simulink model "espectro"  (R2012b)
settings: Solver=ode45  StartTime=0.0  StopTime=10.0  RelTol=1e-3
libraries: xbsIndex_r4 x39, xps_library x25, dspsigops x16, monroe_library x2
settings Model: Creator=root  LastModifiedBy=root

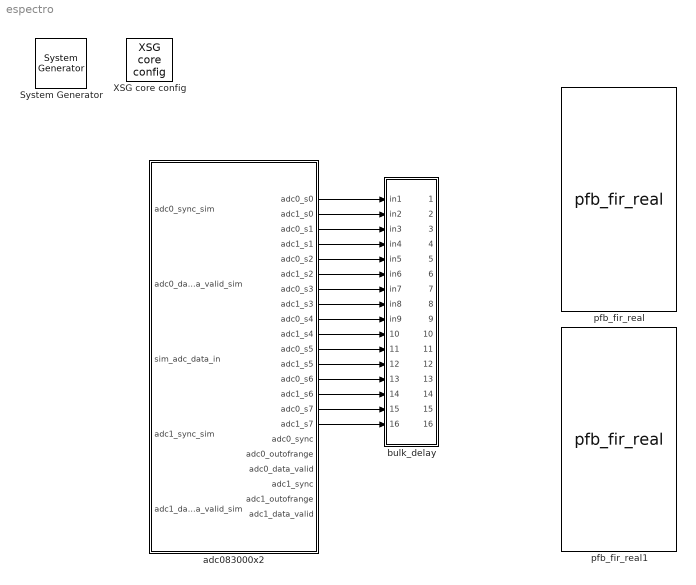
== system espectro ==
  " System Generator" : xbsIndex_r4/ System Generator  Tag=genX  xilinxfamily=virtex5  part=xc5vsx95t  speed=-1  package=ff1136  synthesis_tool=XST  clock_wrapper=Clock Enables  directory=./spec_2pol_4kw_6tap_pfb/sysgen  proj_type=Project Navigator  Synth_file=XST Defaults  Impl_file=ISE Defaults  testbench=off  simulink_period=1  sysclk_period=2.6667  dcm_input_clock_period=100  incr_netlist=off  trim_vbits=Everywhere in SubSystem  dbl_ovrd=According to Block Masks  core_generation=According to Block Masks  run_coregen=off  deprecated_control=off  eval_field=0  block_type=sysgen
      settings: block_version=11.4
  XSG core config : xps_library/XSG core config  Tag=xps:xsg  hw_sys=ROACH:sx95t  clk_src=adc0_clk  ROACH_clk_src=adc0_clk  ROACH2_clk_src=adc0_clk  clk_rate=375  sample_period=1  synthesis_tool=XST
  adc083000x2 : Subsystem  Tag=xps:adc083000x2  AncestorBlock=xps_library/adc083000x2  mask(adc_083000x2){use_adc0=on, use_adc1=on, demux_adc=off, clock_sync=on, verbose=off, using_ctrl=on, adc_clk_rate=1000, sample_period=1, bit_width=8}
      mask prompts: use_adc0 "Use ZD0K0?"; use_adc1 "Use ZDOK1?"; demux_adc "Demux ADCs by 2?"; clock_sync "Interleave 2 ADC boards?"; verbose "Verbose Block Creation?"; using_ctrl "Add ports for control registers?"; adc_clk_rate "ADC clock rate (MHz)"; sample_period "Sample Period"; bit_width "Output Bit Width"
      mask help:
      | The ADC block converts analog inputs to digital outputs.
      | Every clock cycle, the inputs are sampled and digitized to
      | 8 bit binary point numbers in the range of [-1, 1).
      |
      | Online block-specific documentation: http://casper.berkeley.edu/wiki/Adc083000
      mask init:
      | adc083000_mask;
      mask Help: eval('xlWeb([getenv(''MLIB_ROOT''), ''\doc\html\sys_adc\sys_adc.html''])')
  bulk_delay : Subsystem  AncestorBlock=monroe_library/bulk_delay  mask{numInputs=9, delay_arr=5}
      mask prompts: numInputs "# Inputs?"; delay_arr "Delays (integer or array of #inputs elements)"
      mask init:
      | config.source=str2func('bulk_delay_draw');
      | config.toplevel=gcb;
      | config.debug=0;
      | config.depend={'bulk_delay_draw.m'};
      | xBlock(config,{numInputs,delay_arr});
  pfb_fir_real : monroe_library/pfb_fir_real  pfb_size=14  n_sim_inputs=4  n_taps=4  data_n_bits=18  coeff_n_bits=18  output_bit_width=18  window_fn=hamming  bin_width=1  end_scale_val=1  endDelay=off  cheap_sync=off  autoplace_mode='Attached to both ADC0 and ADC1 (interleaved)'  autoplace_optimize=off  bram_latency_coeff=off  bram_latency_delay=off  register_counter=off  pack_delays=on
  pfb_fir_real1 : monroe_library/pfb_fir_real  pfb_size=14  n_sim_inputs=4  n_taps=4  data_n_bits=18  coeff_n_bits=18  output_bit_width=18  window_fn=hamming  bin_width=1  end_scale_val=1  endDelay=off  cheap_sync=off  autoplace_mode='Attached to both ADC0 and ADC1 (interleaved)'  autoplace_optimize=off  bram_latency_coeff=off  bram_latency_delay=off  register_counter=off  pack_delays=on
  wires:
  adc083000x2/1(adc0_s0) -> bulk_delay/1(in1)
  adc083000x2/2(adc1_s0) -> bulk_delay/2(in2)
  adc083000x2/3(adc0_s1) -> bulk_delay/3(in3)
  adc083000x2/4(adc1_s1) -> bulk_delay/4(in4)
  adc083000x2/5(adc0_s2) -> bulk_delay/5(in5)
  adc083000x2/6(adc1_s2) -> bulk_delay/6(in6)
  adc083000x2/7(adc0_s3) -> bulk_delay/7(in7)
  adc083000x2/8(adc1_s3) -> bulk_delay/8(in8)
  adc083000x2/9(adc0_s4) -> bulk_delay/9(in9)
  adc083000x2/10(adc1_s4) -> bulk_delay/10(in10)
  adc083000x2/11(adc0_s5) -> bulk_delay/11(in11)
  adc083000x2/12(adc1_s5) -> bulk_delay/12(in12)
  adc083000x2/13(adc0_s6) -> bulk_delay/13(in13)
  adc083000x2/14(adc1_s6) -> bulk_delay/14(in14)
  adc083000x2/15(adc0_s7) -> bulk_delay/15(in15)
  adc083000x2/16(adc1_s7) -> bulk_delay/16(in16)

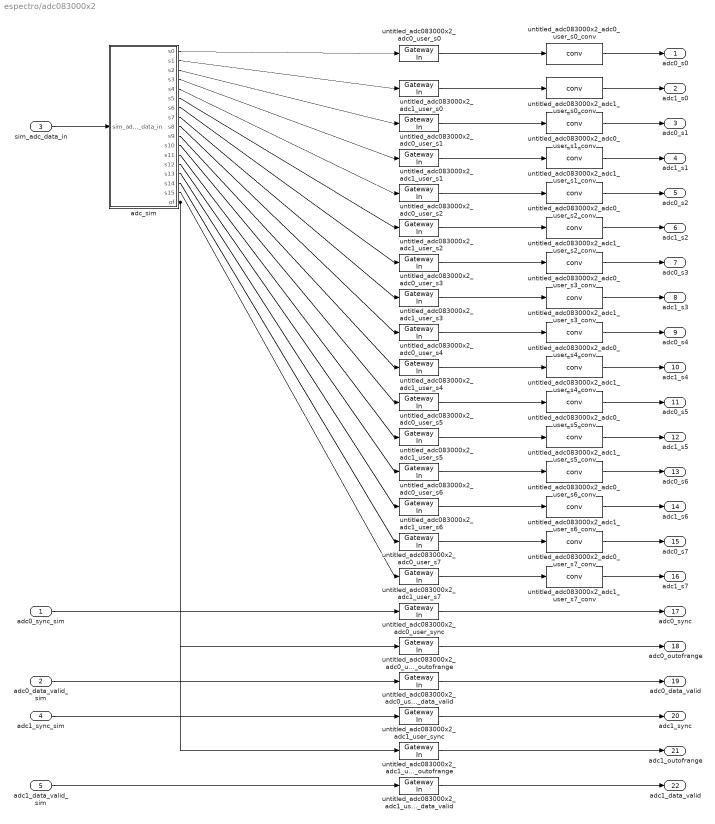
== system espectro/adc083000x2 ==
  adc0_sync_sim : Inport
  adc0_data_valid_sim : Inport  Port=2
  sim_adc_data_in : Inport  Port=3
  adc1_sync_sim : Inport  Port=4
  adc1_data_valid_sim : Inport  Port=5
  adc_sim : Subsystem  AncestorBlock=xps_library/ADCs/adc_sim  mask(adc_sim){nStreams=16, bit_width=8}
      mask prompts: nStreams "Number of Output Streams"; bit_width "Sample Bit Width"
      mask help:
      | This block simulates the behavior of a demuxed ADC, which takes
      | as input a waveform and returns digital samples in parallel at
      | a slower rate.
      |
      | This block is used to simulate the behavior
      mask init:
      | adc_sim_init(gcb, ...
      |     'nStreams', nStreams, ...
      |     'bit_width', bit_width);
  untitled_adc083000x2_adc0_user_data_valid : xbsIndex_r4/Gateway In  gui_display_data_type=Fixed-point  arith_type=Unsigned  n_bits=1  bin_pt=0  preci_type=Single  exp_width=8  frac_width=24  quantization="Round  (unbiased: +/- Inf)"  overflow=Saturate  period=1  dbl_ovrd=off  timing_constraint=None  locs_specified=off  LOCs={}  UseAsADC=off  ADCChannel='1'  inherit_from_input=off  hdl_port=on  block_type=gatewayin
  untitled_adc083000x2_adc0_user_outofrange : xbsIndex_r4/Gateway In  gui_display_data_type=Fixed-point  arith_type=Unsigned  n_bits=4  bin_pt=0  preci_type=Single  exp_width=8  frac_width=24  quantization="Round  (unbiased: +/- Inf)"  overflow=Saturate  period=1  dbl_ovrd=off  timing_constraint=None  locs_specified=off  LOCs={}  UseAsADC=off  ADCChannel='1'  inherit_from_input=off  hdl_port=on  block_type=gatewayin
  untitled_adc083000x2_adc0_user_s{0..7} (8 alike) : xbsIndex_r4/Gateway In  gui_display_data_type=Fixed-point  arith_type=Unsigned  n_bits=8  bin_pt=0  preci_type=Single  exp_width=8  frac_width=24  quantization="Round  (unbiased: +/- Inf)"  overflow=Saturate  period=1  dbl_ovrd=off  timing_constraint=None  locs_specified=off  LOCs={}  UseAsADC=off  ADCChannel='1'  inherit_from_input=off  hdl_port=on  block_type=gatewayin
  untitled_adc083000x2_adc0_user_s0_conv : xps_library/ADCs/conv  bit_width=8
  untitled_adc083000x2_adc0_user_s1_conv : xps_library/ADCs/conv  bit_width=8
  untitled_adc083000x2_adc0_user_s2_conv : xps_library/ADCs/conv  bit_width=8
  untitled_adc083000x2_adc0_user_s3_conv : xps_library/ADCs/conv  bit_width=8
  untitled_adc083000x2_adc0_user_s4_conv : xps_library/ADCs/conv  bit_width=8
  untitled_adc083000x2_adc0_user_s5_conv : xps_library/ADCs/conv  bit_width=8
  untitled_adc083000x2_adc0_user_s6_conv : xps_library/ADCs/conv  bit_width=8
  untitled_adc083000x2_adc0_user_s7_conv : xps_library/ADCs/conv  bit_width=8
  untitled_adc083000x2_adc0_user_sync : xbsIndex_r4/Gateway In  gui_display_data_type=Fixed-point  arith_type=Unsigned  n_bits=4  bin_pt=0  preci_type=Single  exp_width=8  frac_width=24  quantization="Round  (unbiased: +/- Inf)"  overflow=Saturate  period=1  dbl_ovrd=off  timing_constraint=None  locs_specified=off  LOCs={}  UseAsADC=off  ADCChannel='1'  inherit_from_input=off  hdl_port=on  block_type=gatewayin
  untitled_adc083000x2_adc1_user_data_valid : xbsIndex_r4/Gateway In  gui_display_data_type=Fixed-point  arith_type=Unsigned  n_bits=1  bin_pt=0  preci_type=Single  exp_width=8  frac_width=24  quantization="Round  (unbiased: +/- Inf)"  overflow=Saturate  period=1  dbl_ovrd=off  timing_constraint=None  locs_specified=off  LOCs={}  UseAsADC=off  ADCChannel='1'  inherit_from_input=off  hdl_port=on  block_type=gatewayin
  untitled_adc083000x2_adc1_user_outofrange : xbsIndex_r4/Gateway In  gui_display_data_type=Fixed-point  arith_type=Unsigned  n_bits=4  bin_pt=0  preci_type=Single  exp_width=8  frac_width=24  quantization="Round  (unbiased: +/- Inf)"  overflow=Saturate  period=1  dbl_ovrd=off  timing_constraint=None  locs_specified=off  LOCs={}  UseAsADC=off  ADCChannel='1'  inherit_from_input=off  hdl_port=on  block_type=gatewayin
  untitled_adc083000x2_adc1_user_s{0..7} (8 alike) : xbsIndex_r4/Gateway In  gui_display_data_type=Fixed-point  arith_type=Unsigned  n_bits=8  bin_pt=0  preci_type=Single  exp_width=8  frac_width=24  quantization="Round  (unbiased: +/- Inf)"  overflow=Saturate  period=1  dbl_ovrd=off  timing_constraint=None  locs_specified=off  LOCs={}  UseAsADC=off  ADCChannel='1'  inherit_from_input=off  hdl_port=on  block_type=gatewayin
  untitled_adc083000x2_adc1_user_s0_conv : xps_library/ADCs/conv  bit_width=8
  untitled_adc083000x2_adc1_user_s1_conv : xps_library/ADCs/conv  bit_width=8
  untitled_adc083000x2_adc1_user_s2_conv : xps_library/ADCs/conv  bit_width=8
  untitled_adc083000x2_adc1_user_s3_conv : xps_library/ADCs/conv  bit_width=8
  untitled_adc083000x2_adc1_user_s4_conv : xps_library/ADCs/conv  bit_width=8
  untitled_adc083000x2_adc1_user_s5_conv : xps_library/ADCs/conv  bit_width=8
  untitled_adc083000x2_adc1_user_s6_conv : xps_library/ADCs/conv  bit_width=8
  untitled_adc083000x2_adc1_user_s7_conv : xps_library/ADCs/conv  bit_width=8
  untitled_adc083000x2_adc1_user_sync : xbsIndex_r4/Gateway In  gui_display_data_type=Fixed-point  arith_type=Unsigned  n_bits=4  bin_pt=0  preci_type=Single  exp_width=8  frac_width=24  quantization="Round  (unbiased: +/- Inf)"  overflow=Saturate  period=1  dbl_ovrd=off  timing_constraint=None  locs_specified=off  LOCs={}  UseAsADC=off  ADCChannel='1'  inherit_from_input=off  hdl_port=on  block_type=gatewayin
  adc0_s0 : Outport
  adc1_s0 : Outport  Port=2
  adc0_s1 : Outport  Port=3
  adc1_s1 : Outport  Port=4
  adc0_s2 : Outport  Port=5
  adc1_s2 : Outport  Port=6
  adc0_s3 : Outport  Port=7
  adc1_s3 : Outport  Port=8
  adc0_s4 : Outport  Port=9
  adc1_s4 : Outport  Port=10
  adc0_s5 : Outport  Port=11
  adc1_s5 : Outport  Port=12
  adc0_s6 : Outport  Port=13
  adc1_s6 : Outport  Port=14
  adc0_s7 : Outport  Port=15
  adc1_s7 : Outport  Port=16
  adc0_sync : Outport  Port=17
  adc0_outofrange : Outport  Port=18
  adc0_data_valid : Outport  Port=19
  adc1_sync : Outport  Port=20
  adc1_outofrange : Outport  Port=21
  adc1_data_valid : Outport  Port=22
  wires:
  sim_adc_data_in/1 -> adc_sim/1(sim_adc_data_in)
  adc_sim/1(s0) -> untitled_adc083000x2_adc0_user_s0/1
  untitled_adc083000x2_adc0_user_s0/1 -> untitled_adc083000x2_adc0_user_s0_conv/1
  untitled_adc083000x2_adc0_user_s0_conv/1 -> adc0_s0/1
  adc_sim/2(s1) -> untitled_adc083000x2_adc1_user_s0/1
  untitled_adc083000x2_adc1_user_s0/1 -> untitled_adc083000x2_adc1_user_s0_conv/1
  untitled_adc083000x2_adc1_user_s0_conv/1 -> adc1_s0/1
  adc_sim/3(s2) -> untitled_adc083000x2_adc0_user_s1/1
  untitled_adc083000x2_adc0_user_s1/1 -> untitled_adc083000x2_adc0_user_s1_conv/1
  untitled_adc083000x2_adc0_user_s1_conv/1 -> adc0_s1/1
  adc_sim/4(s3) -> untitled_adc083000x2_adc1_user_s1/1
  untitled_adc083000x2_adc1_user_s1/1 -> untitled_adc083000x2_adc1_user_s1_conv/1
  untitled_adc083000x2_adc1_user_s1_conv/1 -> adc1_s1/1
  adc_sim/5(s4) -> untitled_adc083000x2_adc0_user_s2/1
  untitled_adc083000x2_adc0_user_s2/1 -> untitled_adc083000x2_adc0_user_s2_conv/1
  untitled_adc083000x2_adc0_user_s2_conv/1 -> adc0_s2/1
  adc_sim/6(s5) -> untitled_adc083000x2_adc1_user_s2/1
  untitled_adc083000x2_adc1_user_s2/1 -> untitled_adc083000x2_adc1_user_s2_conv/1
  untitled_adc083000x2_adc1_user_s2_conv/1 -> adc1_s2/1
  adc_sim/7(s6) -> untitled_adc083000x2_adc0_user_s3/1
  untitled_adc083000x2_adc0_user_s3/1 -> untitled_adc083000x2_adc0_user_s3_conv/1
  untitled_adc083000x2_adc0_user_s3_conv/1 -> adc0_s3/1
  adc_sim/8(s7) -> untitled_adc083000x2_adc1_user_s3/1
  untitled_adc083000x2_adc1_user_s3/1 -> untitled_adc083000x2_adc1_user_s3_conv/1
  untitled_adc083000x2_adc1_user_s3_conv/1 -> adc1_s3/1
  adc_sim/9(s8) -> untitled_adc083000x2_adc0_user_s4/1
  untitled_adc083000x2_adc0_user_s4/1 -> untitled_adc083000x2_adc0_user_s4_conv/1
  untitled_adc083000x2_adc0_user_s4_conv/1 -> adc0_s4/1
  adc_sim/10(s9) -> untitled_adc083000x2_adc1_user_s4/1
  untitled_adc083000x2_adc1_user_s4/1 -> untitled_adc083000x2_adc1_user_s4_conv/1
  untitled_adc083000x2_adc1_user_s4_conv/1 -> adc1_s4/1
  adc_sim/11(s10) -> untitled_adc083000x2_adc0_user_s5/1
  untitled_adc083000x2_adc0_user_s5/1 -> untitled_adc083000x2_adc0_user_s5_conv/1
  untitled_adc083000x2_adc0_user_s5_conv/1 -> adc0_s5/1
  adc_sim/12(s11) -> untitled_adc083000x2_adc1_user_s5/1
  untitled_adc083000x2_adc1_user_s5/1 -> untitled_adc083000x2_adc1_user_s5_conv/1
  untitled_adc083000x2_adc1_user_s5_conv/1 -> adc1_s5/1
  adc_sim/13(s12) -> untitled_adc083000x2_adc0_user_s6/1
  untitled_adc083000x2_adc0_user_s6/1 -> untitled_adc083000x2_adc0_user_s6_conv/1
  untitled_adc083000x2_adc0_user_s6_conv/1 -> adc0_s6/1
  adc_sim/14(s13) -> untitled_adc083000x2_adc1_user_s6/1
  untitled_adc083000x2_adc1_user_s6/1 -> untitled_adc083000x2_adc1_user_s6_conv/1
  untitled_adc083000x2_adc1_user_s6_conv/1 -> adc1_s6/1
  adc_sim/15(s14) -> untitled_adc083000x2_adc0_user_s7/1
  untitled_adc083000x2_adc0_user_s7/1 -> untitled_adc083000x2_adc0_user_s7_conv/1
  untitled_adc083000x2_adc0_user_s7_conv/1 -> adc0_s7/1
  adc_sim/16(s15) -> untitled_adc083000x2_adc1_user_s7/1
  untitled_adc083000x2_adc1_user_s7/1 -> untitled_adc083000x2_adc1_user_s7_conv/1
  untitled_adc083000x2_adc1_user_s7_conv/1 -> adc1_s7/1
  adc0_sync_sim/1 -> untitled_adc083000x2_adc0_user_sync/1
  untitled_adc083000x2_adc0_user_sync/1 -> adc0_sync/1
  adc_sim/17(of) -> untitled_adc083000x2_adc0_user_outofrange/1, untitled_adc083000x2_adc1_user_outofrange/1
  untitled_adc083000x2_adc0_user_outofrange/1 -> adc0_outofrange/1
  adc0_data_valid_sim/1 -> untitled_adc083000x2_adc0_user_data_valid/1
  untitled_adc083000x2_adc0_user_data_valid/1 -> adc0_data_valid/1
  adc1_sync_sim/1 -> untitled_adc083000x2_adc1_user_sync/1
  untitled_adc083000x2_adc1_user_sync/1 -> adc1_sync/1
  untitled_adc083000x2_adc1_user_outofrange/1 -> adc1_outofrange/1
  adc1_data_valid_sim/1 -> untitled_adc083000x2_adc1_user_data_valid/1
  untitled_adc083000x2_adc1_user_data_valid/1 -> adc1_data_valid/1

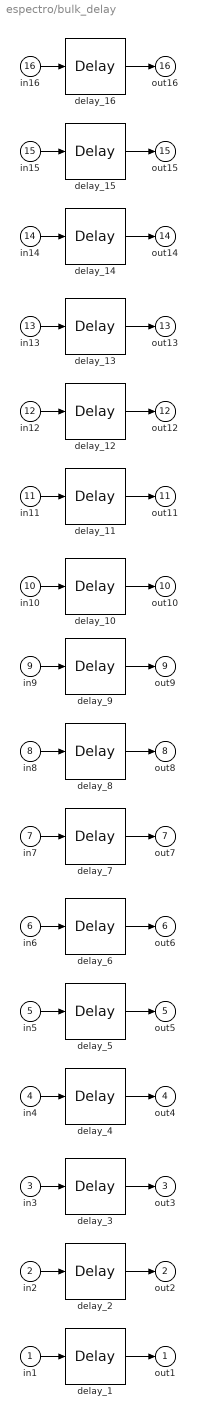
== system espectro/bulk_delay ==
  in1 : Inport
  in2 : Inport  Port=2
  in3 : Inport  Port=3
  in4 : Inport  Port=4
  in5 : Inport  Port=5
  in6 : Inport  Port=6
  in7 : Inport  Port=7
  in8 : Inport  Port=8
  in9 : Inport  Port=9
  in10 : Inport  Port=10
  in11 : Inport  Port=11
  in12 : Inport  Port=12
  in13 : Inport  Port=13
  in14 : Inport  Port=14
  in15 : Inport  Port=15
  in16 : Inport  Port=16
  delay_{1..16} (16 alike) : xbsIndex_r4/Delay  rst=off  infoeditControl=Selection of Reset will increase slice count due to use of real FFs and instead of SRLs  en=off  latency=5  dbl_ovrd=off  reg_retiming=off  block_type=delay
  out1 : Outport
  out2 : Outport  Port=2
  out3 : Outport  Port=3
  out4 : Outport  Port=4
  out5 : Outport  Port=5
  out6 : Outport  Port=6
  out7 : Outport  Port=7
  out8 : Outport  Port=8
  out9 : Outport  Port=9
  out10 : Outport  Port=10
  out11 : Outport  Port=11
  out12 : Outport  Port=12
  out13 : Outport  Port=13
  out14 : Outport  Port=14
  out15 : Outport  Port=15
  out16 : Outport  Port=16
  wires:
  in1/1 -> delay_1/1
  delay_1/1 -> out1/1
  in2/1 -> delay_2/1
  delay_2/1 -> out2/1
  in3/1 -> delay_3/1
  delay_3/1 -> out3/1
  in4/1 -> delay_4/1
  delay_4/1 -> out4/1
  in5/1 -> delay_5/1
  delay_5/1 -> out5/1
  in6/1 -> delay_6/1
  delay_6/1 -> out6/1
  in7/1 -> delay_7/1
  delay_7/1 -> out7/1
  in8/1 -> delay_8/1
  delay_8/1 -> out8/1
  in9/1 -> delay_9/1
  delay_9/1 -> out9/1
  in10/1 -> delay_10/1
  delay_10/1 -> out10/1
  in11/1 -> delay_11/1
  delay_11/1 -> out11/1
  in12/1 -> delay_12/1
  delay_12/1 -> out12/1
  in13/1 -> delay_13/1
  delay_13/1 -> out13/1
  in14/1 -> delay_14/1
  delay_14/1 -> out14/1
  in15/1 -> delay_15/1
  delay_15/1 -> out15/1
  in16/1 -> delay_16/1
  delay_16/1 -> out16/1

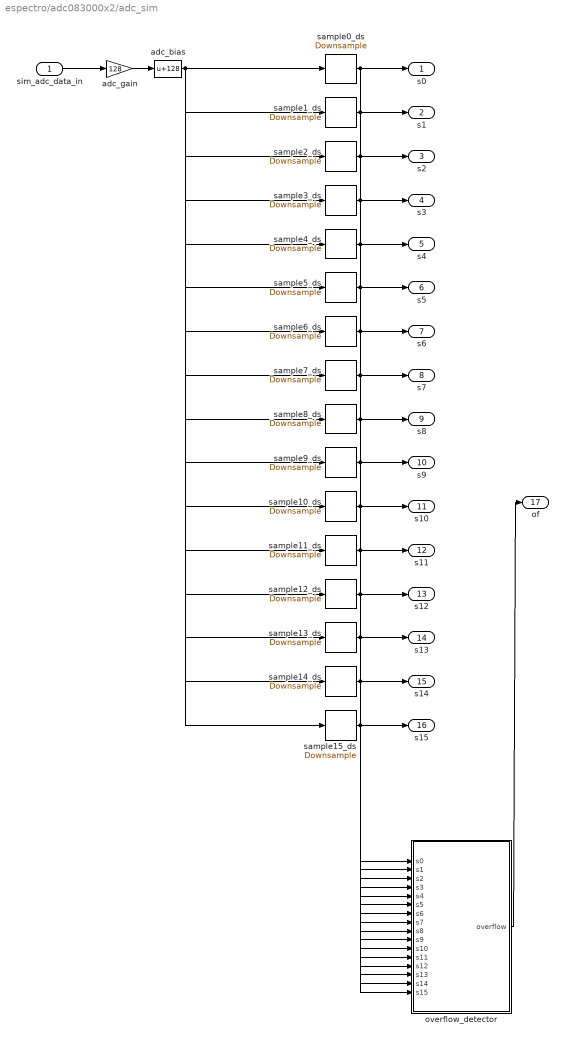
== system espectro/adc083000x2/adc_sim ==
  sim_adc_data_in : Inport
  adc_bias : Bias  Bias=128  SaturateOnIntegerOverflow=on
  adc_gain : Gain  Gain=128
  overflow_detector : Subsystem  AncestorBlock=xps_library/ADCs/of_detect_bus  mask(of_detect_bus){nStreams=16, bit_width=8}
      mask prompts: nStreams "Number of Streams"; bit_width "Bit Width"
      mask init:
      | of_detect_bus_init(gcb, ...
      |     'nStreams', nStreams, ...
      |     'bit_width', bit_width);
  sample0_ds : dspsigops/Downsample  N=16  phase=1  InputProcessing=Inherited (this choice will be removed - see release notes)  RateOptions=Enforce single-rate processing  smode=Force single rate  fmode=Maintain input frame rate  ic=0
  sample10_ds : dspsigops/Downsample  N=16  phase=11  InputProcessing=Inherited (this choice will be removed - see release notes)  RateOptions=Enforce single-rate processing  smode=Force single rate  fmode=Maintain input frame rate  ic=0
  sample11_ds : dspsigops/Downsample  N=16  phase=12  InputProcessing=Inherited (this choice will be removed - see release notes)  RateOptions=Enforce single-rate processing  smode=Force single rate  fmode=Maintain input frame rate  ic=0
  sample12_ds : dspsigops/Downsample  N=16  phase=13  InputProcessing=Inherited (this choice will be removed - see release notes)  RateOptions=Enforce single-rate processing  smode=Force single rate  fmode=Maintain input frame rate  ic=0
  sample13_ds : dspsigops/Downsample  N=16  phase=14  InputProcessing=Inherited (this choice will be removed - see release notes)  RateOptions=Enforce single-rate processing  smode=Force single rate  fmode=Maintain input frame rate  ic=0
  sample14_ds : dspsigops/Downsample  N=16  phase=15  InputProcessing=Inherited (this choice will be removed - see release notes)  RateOptions=Enforce single-rate processing  smode=Force single rate  fmode=Maintain input frame rate  ic=0
  sample15_ds : dspsigops/Downsample  N=16  phase=0  InputProcessing=Inherited (this choice will be removed - see release notes)  RateOptions=Enforce single-rate processing  smode=Force single rate  fmode=Maintain input frame rate  ic=0
  sample1_ds : dspsigops/Downsample  N=16  phase=2  InputProcessing=Inherited (this choice will be removed - see release notes)  RateOptions=Enforce single-rate processing  smode=Force single rate  fmode=Maintain input frame rate  ic=0
  sample2_ds : dspsigops/Downsample  N=16  phase=3  InputProcessing=Inherited (this choice will be removed - see release notes)  RateOptions=Enforce single-rate processing  smode=Force single rate  fmode=Maintain input frame rate  ic=0
  sample3_ds : dspsigops/Downsample  N=16  phase=4  InputProcessing=Inherited (this choice will be removed - see release notes)  RateOptions=Enforce single-rate processing  smode=Force single rate  fmode=Maintain input frame rate  ic=0
  sample4_ds : dspsigops/Downsample  N=16  phase=5  InputProcessing=Inherited (this choice will be removed - see release notes)  RateOptions=Enforce single-rate processing  smode=Force single rate  fmode=Maintain input frame rate  ic=0
  sample5_ds : dspsigops/Downsample  N=16  phase=6  InputProcessing=Inherited (this choice will be removed - see release notes)  RateOptions=Enforce single-rate processing  smode=Force single rate  fmode=Maintain input frame rate  ic=0
  sample6_ds : dspsigops/Downsample  N=16  phase=7  InputProcessing=Inherited (this choice will be removed - see release notes)  RateOptions=Enforce single-rate processing  smode=Force single rate  fmode=Maintain input frame rate  ic=0
  sample7_ds : dspsigops/Downsample  N=16  phase=8  InputProcessing=Inherited (this choice will be removed - see release notes)  RateOptions=Enforce single-rate processing  smode=Force single rate  fmode=Maintain input frame rate  ic=0
  sample8_ds : dspsigops/Downsample  N=16  phase=9  InputProcessing=Inherited (this choice will be removed - see release notes)  RateOptions=Enforce single-rate processing  smode=Force single rate  fmode=Maintain input frame rate  ic=0
  sample9_ds : dspsigops/Downsample  N=16  phase=10  InputProcessing=Inherited (this choice will be removed - see release notes)  RateOptions=Enforce single-rate processing  smode=Force single rate  fmode=Maintain input frame rate  ic=0
  s0 : Outport
  s1 : Outport  Port=2
  s2 : Outport  Port=3
  s3 : Outport  Port=4
  s4 : Outport  Port=5
  s5 : Outport  Port=6
  s6 : Outport  Port=7
  s7 : Outport  Port=8
  s8 : Outport  Port=9
  s9 : Outport  Port=10
  s10 : Outport  Port=11
  s11 : Outport  Port=12
  s12 : Outport  Port=13
  s13 : Outport  Port=14
  s14 : Outport  Port=15
  s15 : Outport  Port=16
  of : Outport  Port=17
  wires:
  sim_adc_data_in/1 -> adc_gain/1
  adc_gain/1 -> adc_bias/1
  overflow_detector/1(overflow) -> of/1
  adc_bias/1 -> sample0_ds/1, sample1_ds/1, sample2_ds/1, sample3_ds/1, sample4_ds/1, sample5_ds/1, sample6_ds/1, sample7_ds/1, sample8_ds/1, sample9_ds/1, sample10_ds/1, sample11_ds/1, sample12_ds/1, sample13_ds/1, sample14_ds/1, sample15_ds/1
  sample0_ds/1 -> overflow_detector/1(s0), s0/1
  sample1_ds/1 -> overflow_detector/2(s1), s1/1
  sample2_ds/1 -> overflow_detector/3(s2), s2/1
  sample3_ds/1 -> overflow_detector/4(s3), s3/1
  sample4_ds/1 -> overflow_detector/5(s4), s4/1
  sample5_ds/1 -> overflow_detector/6(s5), s5/1
  sample6_ds/1 -> overflow_detector/7(s6), s6/1
  sample7_ds/1 -> overflow_detector/8(s7), s7/1
  sample8_ds/1 -> overflow_detector/9(s8), s8/1
  sample9_ds/1 -> overflow_detector/10(s9), s9/1
  sample10_ds/1 -> overflow_detector/11(s10), s10/1
  sample11_ds/1 -> overflow_detector/12(s11), s11/1
  sample12_ds/1 -> overflow_detector/13(s12), s12/1
  sample13_ds/1 -> overflow_detector/14(s13), s13/1
  sample14_ds/1 -> overflow_detector/15(s14), s14/1
  sample15_ds/1 -> overflow_detector/16(s15), s15/1

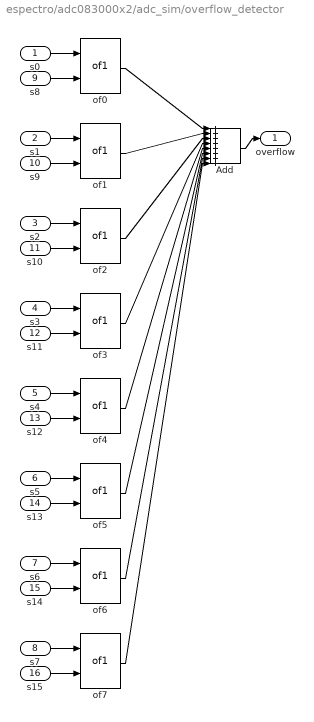
== system espectro/adc083000x2/adc_sim/overflow_detector ==
  s0 : Inport
  s1 : Inport  Port=2
  s2 : Inport  Port=3
  s3 : Inport  Port=4
  s4 : Inport  Port=5
  s5 : Inport  Port=6
  s6 : Inport  Port=7
  s7 : Inport  Port=8
  s8 : Inport  Port=9
  s9 : Inport  Port=10
  s10 : Inport  Port=11
  s11 : Inport  Port=12
  s12 : Inport  Port=13
  s13 : Inport  Port=14
  s14 : Inport  Port=15
  s15 : Inport  Port=16
  Add : Sum  Inputs=++++++++
  of{0..7} (8 alike) : xps_library/ADCs/of1  bit_num=0  n_adc_bits=8
  overflow : Outport
  wires:
  s0/1 -> of0/1
  s8/1 -> of0/2
  of0/1 -> Add/1
  s1/1 -> of1/1
  s9/1 -> of1/2
  of1/1 -> Add/2
  s2/1 -> of2/1
  s10/1 -> of2/2
  of2/1 -> Add/3
  s3/1 -> of3/1
  s11/1 -> of3/2
  of3/1 -> Add/4
  s4/1 -> of4/1
  s12/1 -> of4/2
  of4/1 -> Add/5
  s5/1 -> of5/1
  s13/1 -> of5/2
  of5/1 -> Add/6
  s6/1 -> of6/1
  s14/1 -> of6/2
  of6/1 -> Add/7
  s7/1 -> of7/1
  s15/1 -> of7/2
  of7/1 -> Add/8
  Add/1 -> overflow/1
